simulink model "arduino_serial_gps"  (R2021b)
settings: Solver=FixedStepAuto  StartTime=0.0  StopTime=10  RelTol=1e-3
PreLoadFcn:
  | addpath(fullfile(fileparts(codertarget.arduinobase.internal.getBaseSpPkgRootDir), 'arduinotarget', 'arduinotargetdemos','demo_src'));
libraries: arduinolib x1, realtime_examples_misc x1
CloseFcn:
  | if (exist('GPSParser.m', 'file') == 2)
  | rmpath(fullfile(fileparts(codertarget.arduinobase.internal.getBaseSpPkgRootDir), 'arduinotarget', 'arduinotargetdemos','demo_src'));
  | end
settings Model: SimulationMode=external  ExtModeTrigDuration=2  ExtModeArchiveDirName=C:\Users\mmordeka\Desktop\2_6_morning  ExtModeAddSuffixToVar=on  Creator=The MathWorks, Inc.  LastModifiedBy=The MathWorks, Inc.
settings SolverCC: AlgebraicLoopSolver=TrustRegion
settings DataIOCC: ReturnWorkspaceOutputs=off
settings OptimizationCC: PassReuseOutputArgsThreshold=0  MaxStackSize=64
settings DebuggingCC: ParameterTunabilityLossMsg=error  SFMachineParentedDataDiag=warning  ArithmeticOperatorsInVariantConditions=warning
settings HardwareCC: ProdBitPerInt=16  ProdBitPerPointer=16  ProdBitPerSizeT=16  ProdBitPerPtrDiffT=16  ProdLargestAtomicFloat=None  ProdWordSize=8  ProdHWDeviceType=Atmel->AVR  UseEmbeddedCoderFeatures=off  UseSimulinkCoderFeatures=off
settings SFSimCC: SimUseLocalCustomCode=off  MATLABDynamicMemAlloc=off
settings RTWCC: Description=Embedded Coder  SystemTargetFile=ert.tlc  HardwareBoard=Arduino Mega 2560  TemplateMakefile=ert_default_tmf  GenerateReport=on  RTWUseLocalCustomCode=off  Toolchain=Arduino AVR  BuildConfiguration=Faster Runs  LaunchReport=on
settings CodeAppCC: ForceParamTrailComments=on  OperatorAnnotations=on  StateflowObjectComments=on  MATLABSourceComments=on
settings ERTTargetCC: ERTCustomFileBanners=off  SupportContinuousTime=on  SupportNonInlinedSFcns=on  RemoveResetFunc=off  SupportVariableSizeSignals=on  ModelStepFunctionPrototypeControlCompliant=off

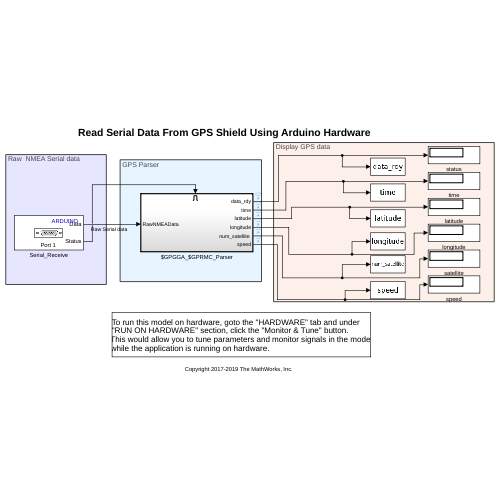
[thumbnail: Simulink's stored preview of the top-level diagram]
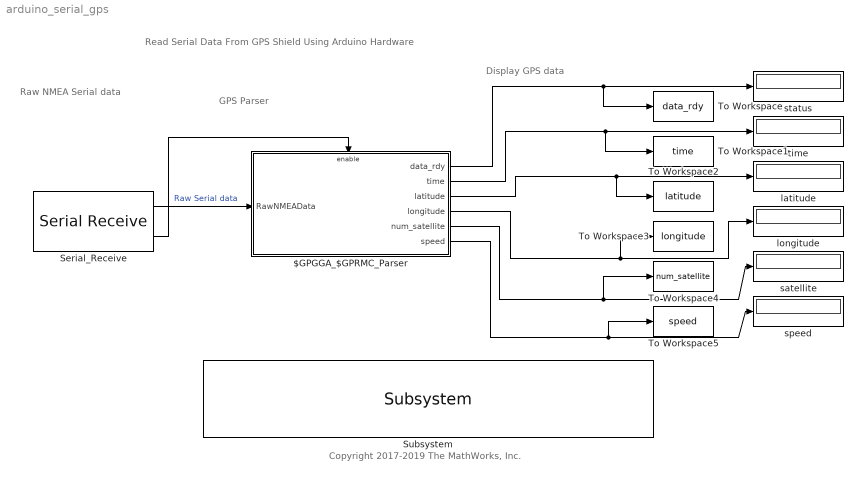
== system arduino_serial_gps ==
  note: Display GPS data
  note: GPS Parser
  note: Raw NMEA Serial data
  note: Read Serial Data From GPS Shield Using Arduino Hardware
  note: Copyright 2017-2019 The MathWorks, Inc.
  $GPGGA_$GPRMC_Parser : Subsystem  TreatAsAtomicUnit=on
  Serial_Receive : arduinolib/Serial Receive  isARMArch=off  portNumber=1  DataType=uint8  Datalength=32  SampleTime=0.03  showOutStatus=on  blockPlatform=arduino
      settings: SourceProductBaseCode=ARDUINO
  Subsystem : realtime_examples_misc/Subsystem  SystemSampleTime=-1  VariantActivationTime=update diagram  Latency=0  AutoFrameSizeCalculation=off
      settings: SourceProductBaseCode=SL
  To Workspace : ToWorkspace  VariableName=data_rdy  SampleTime=-1
      settings: Save2DSignal=2-D array (concatenate along first dimension)
  To Workspace1 : ToWorkspace  VariableName=time  SampleTime=-1
      settings: Save2DSignal=2-D array (concatenate along first dimension)
  To Workspace2 : ToWorkspace  VariableName=latitude  SampleTime=-1
      settings: Save2DSignal=2-D array (concatenate along first dimension)
  To Workspace3 : ToWorkspace  VariableName=longitude  SampleTime=-1
      settings: Save2DSignal=2-D array (concatenate along first dimension)
  To Workspace4 : ToWorkspace  VariableName=num_satellite  SampleTime=-1
      settings: Save2DSignal=2-D array (concatenate along first dimension)
  To Workspace5 : ToWorkspace  VariableName=speed  SampleTime=-1
      settings: Save2DSignal=2-D array (concatenate along first dimension)
  latitude : Display
  longitude : Display
  satellite : Display
  speed : Display
  status : Display
  time : Display
  wires:
  Serial_Receive/1 -> $GPGGA_$GPRMC_Parser/1(RawNMEAData)  "Raw Serial data"
  Serial_Receive/2 -> $GPGGA_$GPRMC_Parser/Enable
  $GPGGA_$GPRMC_Parser/3(latitude) -> latitude/1, To Workspace2/1
  $GPGGA_$GPRMC_Parser/1(data_rdy) -> status/1, To Workspace/1
  $GPGGA_$GPRMC_Parser/6(speed) -> To Workspace5/1, speed/1
  $GPGGA_$GPRMC_Parser/2(time) -> To Workspace1/1, time/1
  $GPGGA_$GPRMC_Parser/5("num_satellite ") -> To Workspace4/1, satellite/1
  $GPGGA_$GPRMC_Parser/4(longitude) -> longitude/1, To Workspace3/1

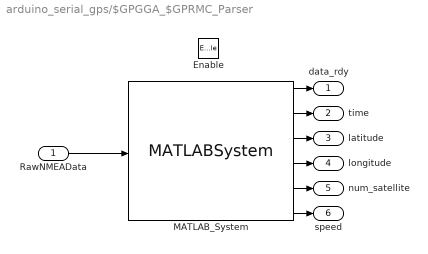
== system arduino_serial_gps/$GPGGA_$GPRMC_Parser ==
  RawNMEAData : Inport
  Enable : EnablePort  StatesWhenEnabling=reset
  MATLAB_System : MATLABSystem  System=GPSParser  TimeOpt=on  LatOpt=on  LonOpt=on  NoSatOpt=on  HdopOpt=off  AltOpt=off  MslOpt=off  SpeedOpt=on  DateOpt=off  TckAngOpt=off
      mask Type: GPSParser
      mask Display:
      | disp('GPSParser');
      | port_label('input',1,'inData');
      | port_label('output',1,'Status');
      | port_label('output',2,'Time');
      | port_label('output',3,'Latitude');
      | port_label('output',4,'Longitude');
      | port_label('output',5,'Satellite');
      | port_label('output',6,'Speed');
  data_rdy : Outport  OutputWhenDisabled=reset  InitialOutput=0  VectorParamsAs1DForOutWhenUnconnected=off
  time : Outport  Port=2  OutputWhenDisabled=reset  InitialOutput=0  VectorParamsAs1DForOutWhenUnconnected=off
  latitude : Outport  Port=3  OutputWhenDisabled=reset  InitialOutput=0  VectorParamsAs1DForOutWhenUnconnected=off
  longitude : Outport  Port=4  OutputWhenDisabled=reset  InitialOutput=0  VectorParamsAs1DForOutWhenUnconnected=off
  "num_satellite " : Outport  Port=5  OutputWhenDisabled=reset  InitialOutput=0  VectorParamsAs1DForOutWhenUnconnected=off
  speed : Outport  Port=6  OutputWhenDisabled=reset  InitialOutput=0  VectorParamsAs1DForOutWhenUnconnected=off
  wires:
  MATLAB_System/1 -> data_rdy/1
  RawNMEAData/1 -> MATLAB_System/1
  MATLAB_System/2 -> time/1
  MATLAB_System/3 -> latitude/1
  MATLAB_System/4 -> longitude/1
  MATLAB_System/5 -> "num_satellite "/1
  MATLAB_System/6 -> speed/1
